simulink model "plclogging"  (R2016a)
settings: Solver=VariableStepAuto  StartTime=0.0  StopTime=600  RelTol=1e-3
PreLoadFcn:
  | addpath('sutils\RealTimeSlower')
InitFcn:
  | Ts_base = 0.5; % seconds
StopFcn:
  | date_string = datestr(now,'yyyymmdd-HHMM');
  | save(['E:\TESTBED_MEASUREMENTS\LFSR\sim_out' date_string '.mat'],'sim_out')
libraries: utility x1, TcAdsLib x1
settings Model: Creator=sensor  LastModifiedBy=sensor
settings GRTTargetCC: GeneratePreprocessorConditionals=Use local settings

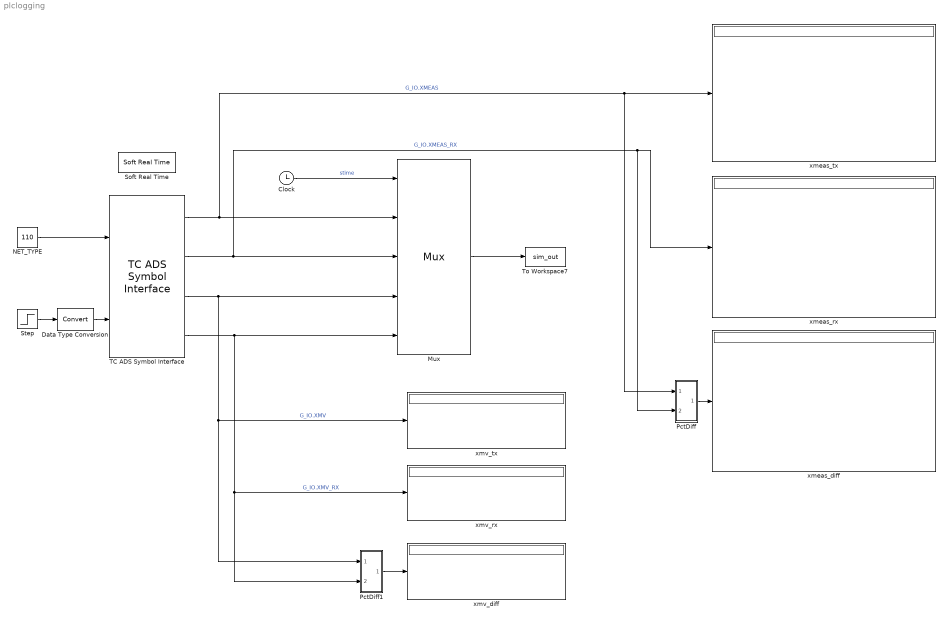
== system plclogging ==
  Clock : Clock
  Data Type Conversion : DataTypeConversion  RndMeth=Round
  Mux : Mux  Inputs=5
      settings: DisplayOption=signals
  NET_TYPE : Constant  Value=110  OutDataTypeStr=int32
  PctDiff : Subsystem
  PctDiff1 : Subsystem
  Soft Real Time : utility/Soft Real Time  x=1
  Step : Step  Time=2  SampleTime=0
      settings: AttributesFormatString=%<Time>
  TC ADS Symbol Interface : TcAdsLib/Synchronous/TC ADS Symbol Interface  ConnectMode=1  TmiPathStorageMode=0  TargetAmsNetId=0.0.0.0.0.0  TargetModuleOid=0  SyncMode=0  TcTimeOutport=0  TimeStampOutport=0  SampleTime=0.25  BufferLength=2  DelayTime=-1  Symbols_SimulinkToTwinCat=|  Symbols_TwinCatToSimulink=|  AdsErrorHandling=2  ChangeRowColOrder=on  CodeGenInputConnectType=DataArea (InputDst)  CodeGenOutputConnectType=DataArea (OutputSrc)
      Symbols_SimulinkToTwinCat=|
      | <?xml version="1.0" encoding="utf-8"?>
      | <SymbolAcquisitionInfoCollection xmlns:xsd="http://www.w3.org/2001/XMLSchema" xmlns:xsi="http://www.w3.org/2001/XMLSchema-instance">
      |   <SymbolInfos>
      |     <SymbolAcquisitionInfo>
      |       <Comment> specify network type
      |  100 					: ISA110.11a iMesh calibration
      |  101 					: ISA110.11a iMesh TESIM
      |  102 					: ISA110.11a iMesh test signals
      |  110					: ISA100.11a iMesh PN Sequence generation
      |  200 					: PhoenixContact calibration
      |  201					: PhoenixContact TESIM
      |  202					: PhoenixContact test signals
      |  210					: ISA100.11a PC OneLink PN Sequence generation</Comment>
      |       <Scope2Datatype>INT32</Scope2Datatype>
      |       <IndexGroup>16448</IndexGroup>
      |       <IndexOffset>593452</IndexOffset>
      |       <Name>G_IO.NET_TYPE</Name>
      |       <ShortName>NET_TYPE</ShortName>
      |       <Size>4</Size>
      |       <Type>DINT</Type>
      |       <TypeGUID>00000000-0000-0000-0000-000000000000</TypeGUID>
      |       <IsArray>false</IsArray>
      |       <ArrayLength>0</ArrayLength>
      |       <ConnectType>Symobl</ConnectType>
      |       <Datatype>ADST_INT32</Datatype>
      |       <NetId>5.20.215.224.1.1</NetId>
      |       <Port>851</Port>
      |       <SubSymbolCount>0</SubSymbolCount>
      |       <IsBitValue>false</IsBitValue>
      |       <IsPersistent>false</IsPersistent>
      |       <IsPointer>false</IsPointer>
      |       <IsReadOnly>false</IsReadOnly>
      |       <IsReference>false</IsReference>
      |       <IsTcComInterfacePointer>false</IsTcComInterfacePointer>
      |       <IsTypeGuid>false</IsTypeGuid>
      |       <ContextMask>0</ContextMask>
      |     </SymbolAcquisitionInfo>
      |     <SymbolAcquisitionInfo>
      |       <Comment />
      |       <Scope2Datatype>BIT</Scope2Datatype>
      |       <IndexGroup>16448</IndexGroup>
      |       <IndexOffset>538604</IndexOffset>
      |       <Name>G_IO.GO</Name>
      |       <ShortName>GO</ShortName>
      |       <Size>1</Size>
      |       <Type>BOOL</Type>
      |       <TypeGUID>00000000-0000-0000-0000-000000000000</TypeGUID>
      |       <IsArray>false</IsArray>
      |       <ArrayLength>0</ArrayLength>
      |       <ConnectType>Symobl</ConnectType>
      |       <Datatype>ADST_BIT</Datatype>
      |       <NetId>5.20.215.224.1.1</NetId>
      |       <Port>851</Port>
      |       <SubSymbolCount>0</SubSymbolCount>
      |       <IsBitValue>false</IsBitValue>
      |       <IsPersistent>false</IsPersistent>
      |       <IsPointer>false</IsPointer>
      |       <IsReadOnly>false</IsReadOnly>
      |       <IsReference>false</IsReference>
      |       <IsTcComInterfacePointer>false</IsTcComInterfacePointer>
      |       <IsTypeGuid>false</IsTypeGuid>
      |       <ContextMask>0</ContextMask>
      |     </SymbolAcquisitionInfo>
      |   </SymbolInfos>
      | </SymbolAcquisitionInfoCollection>
      Symbols_TwinCatToSimulink=|
      | <?xml version="1.0" encoding="utf-8"?>
      | <SymbolAcquisitionInfoCollection xmlns:xsd="http://www.w3.org/2001/XMLSchema" xmlns:xsi="http://www.w3.org/2001/XMLSchema-instance">
      |   <SymbolInfos>
      |     <SymbolAcquisitionInfo>
      |       <Comment> XMEAS reported by tesim</Comment>
      |       <Scope2Datatype>REAL64</Scope2Datatype>
      |       <IndexGroup>16448</IndexGroup>
      |       <IndexOffset>593568</IndexOffset>
      |       <Name>G_IO.XMEAS</Name>
      |       <ShortName>XMEAS</ShortName>
      |       <Size>328</Size>
      |       <Type>ARRAY [1..41] OF LREAL</Type>
      |       <TypeGUID>00000000-0000-0000-0000-000000000000</TypeGUID>
      |       <IsArray>true</IsArray>
      |       <ArrayLength>41</ArrayLength>
      |       <ConnectType>Symobl</ConnectType>
      |       <Datatype>ADST_REAL64</Datatype>
      |       <NetId>5.20.215.224.1.1</NetId>
      |       <Port>851</Port>
      |       <SubSymbolCount>0</SubSymbolCount>
      |       <IsBitValue>false</IsBitValue>
      |       <IsPersistent>false</IsPersistent>
      |       <IsPointer>false</IsPointer>
      |       <IsReadOnly>false</IsReadOnly>
      |       <IsReference>false</IsReference>
      |       <IsTcComInterfacePointer>false</IsTcComInterfacePointer>
      |       <IsTypeGuid>false</IsTypeGuid>
      |       <ContextMask>0</ContextMask>
      |     </SymbolAcquisitionInfo>
      |     <SymbolAcquisitionInfo>
      |       <Comment />
      |       <Scope2Datatype>REAL64</Scope2Datatype>
      |       <IndexGroup>16448</IndexGroup>
      |       <IndexOffset>538768</IndexOffset>
      |       <Name>G_IO.XMEAS_RX</Name>
      |       <ShortName>XMEAS_RX</ShortName>
      |       <Size>328</Size>
      |       <Type>ARRAY [1..41] OF LREAL</Type>
      |       <TypeGUID>00000000-0000-0000-0000-000000000000</TypeGUID>
      |       <IsArray>true</IsArray>
      |       <ArrayLength>41</ArrayLength>
      |       <ConnectType>Symobl</ConnectType>
      |       <Datatype>ADST_REAL64</Datatype>
      |       <NetId>5.20.215.224.1.1</NetId>
      |       <Port>851</Port>
      |       <SubSymbolCount>0</SubSymbolCount>
      |       <IsBitValue>false</IsBitValue>
      |       <IsPersistent>false</IsPersistent>
      |       <IsPointer>false</IsPointer>
      |       <IsReadOnly>false</IsReadOnly>
      |       <IsReference>false</IsReference>
      |       <IsTcComInterfacePointer>false</IsTcComInterfacePointer>
      |       <IsTypeGuid>false</IsTypeGuid>
      |       <ContextMask>0</ContextMask>
      |     </SymbolAcquisitionInfo>
      |     <SymbolAcquisitionInfo>
      |       <Comment> XMV values reported by tesim</Comment>
      |       <Scope2Datatype>REAL64</Scope2Datatype>
      |       <IndexGroup>16448</IndexGroup>
      |       <IndexOffset>593944</IndexOffset>
      |       <Name>G_IO.XMV</Name>
      |       <ShortName>XMV</ShortName>
      |       <Size>96</Size>
      |       <Type>ARRAY [1..12] OF LREAL</Type>
      |       <TypeGUID>00000000-0000-0000-0000-000000000000</TypeGUID>
      |       <IsArray>true</IsArray>
      |       <ArrayLength>12</ArrayLength>
      |       <ConnectType>Symobl</ConnectType>
      |       <Datatype>ADST_REAL64</Datatype>
      |       <NetId>5.20.215.224.1.1</NetId>
      |       <Port>851</Port>
      |       <SubSymbolCount>0</SubSymbolCount>
      |       <IsBitValue>false</IsBitValue>
      |       <IsPersistent>false</IsPersistent>
      |       <IsPointer>false</IsPointer>
      |       <IsReadOnly>false</IsReadOnly>
      |       <IsReference>false</IsReference>
      |       <IsTcComInterfacePointer>false</IsTcComInterfacePointer>
      |       <IsTypeGuid>false</IsTypeGuid>
      |       <ContextMask>0</ContextMask>
      |     </SymbolAcquisitionInfo>
      |     <SymbolAcquisitionInfo>
      |       <Comment />
      |       <Scope2Datatype>REAL64</Scope2Datatype>
      |       <IndexGroup>16448</IndexGroup>
      |       <IndexOffset>540440</IndexOffset>
      |       <Name>G_IO.XMV_RX</Name>
      |       <ShortName>XMV_RX</ShortName>
      |       <Size>96</Size>
      |       <Type>ARRAY [1..12] OF LREAL</Type>
      |       <TypeGUID>00000000-0000-0000-0000-000000000000</TypeGUID>
      |       <IsArray>true</IsArray>
      |       <ArrayLength>12</ArrayLength>
      |       <ConnectType>Symobl</ConnectType>
      |       <Datatype>ADST_REAL64</Datatype>
      |       <NetId>5.20.215.224.1.1</NetId>
      |       <Port>851</Port>
      |       <SubSymbolCount>0</SubSymbolCount>
      |       <IsBitValue>false</IsBitValue>
      |       <IsPersistent>false</IsPersistent>
      |       <IsPointer>false</IsPointer>
      |       <IsReadOnly>false</IsReadOnly>
      |       <IsReference>false</IsReference>
      |       <IsTcComInterfacePointer>false</IsTcComInterfacePointer>
      |       <IsTypeGuid>false</IsTypeGuid>
      |       <ContextMask>0</ContextMask>
      |     </SymbolAcquisitionInfo>
      |   </SymbolInfos>
      | </SymbolAcquisitionInfoCollection>
  To Workspace7 : ToWorkspace  VariableName=sim_out  SampleTime=Ts_base
  xmeas_diff : Display
  xmeas_rx : Display
  xmeas_tx : Display
  xmv_diff : Display
  xmv_rx : Display
  xmv_tx : Display
  wires:
  TC ADS Symbol Interface/3 -> PctDiff1/1(In1), xmv_tx/1, Mux/4  "G_IO.XMV"
  Clock/1 -> Mux/1  "stime"
  TC ADS Symbol Interface/4 -> PctDiff1/2(In2), xmv_rx/1, Mux/5  "G_IO.XMV_RX"
  Mux/1 -> To Workspace7/1
  TC ADS Symbol Interface/2 -> PctDiff/2(In2), xmeas_rx/1, Mux/3  "G_IO.XMEAS_RX"
  TC ADS Symbol Interface/1 -> PctDiff/1(In1), xmeas_tx/1, Mux/2  "G_IO.XMEAS"
  PctDiff/1(Out1) -> xmeas_diff/1
  PctDiff1/1(Out1) -> xmv_diff/1
  NET_TYPE/1 -> TC ADS Symbol Interface/1
  Step/1 -> Data Type Conversion/1
  Data Type Conversion/1 -> TC ADS Symbol Interface/2

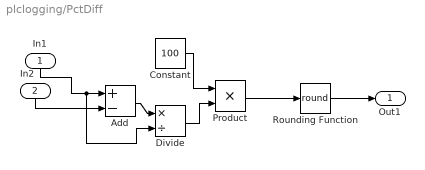
== system plclogging/PctDiff ==
  In1 : Inport
  In2 : Inport  Port=2
  Add : Sum  Inputs=+-
  Constant : Constant  Value=100
  Divide : Product  Inputs=*/
  Product : Product
  Rounding Function : Rounding  Operator=round
  Out1 : Outport
  wires:
  In1/1 -> Divide/2, Add/1
  In2/1 -> Add/2
  Add/1 -> Divide/1
  Constant/1 -> Product/1
  Product/1 -> Rounding Function/1
  Divide/1 -> Product/2
  Rounding Function/1 -> Out1/1

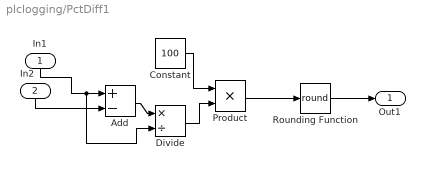
== system plclogging/PctDiff1 ==
  In1 : Inport
  In2 : Inport  Port=2
  Add : Sum  Inputs=+-
  Constant : Constant  Value=100
  Divide : Product  Inputs=*/
  Product : Product
  Rounding Function : Rounding  Operator=round
  Out1 : Outport
  wires:
  In1/1 -> Divide/2, Add/1
  In2/1 -> Add/2
  Add/1 -> Divide/1
  Constant/1 -> Product/1
  Product/1 -> Rounding Function/1
  Divide/1 -> Product/2
  Rounding Function/1 -> Out1/1
